simulink library "Ventilation"  (R2018b)
settings: Solver=ode45  StartTime=0.0  StopTime=10.0  RelTol=1e-3  EnableMultiTasking=on
libraries: carnot x4
settings Model: Creator=lena.frank  LastModifiedBy=drhf
settings DataIOCC: LimitDataPoints=on  SaveFormat=Array  SignalLoggingSaveFormat=ModelDataLogs
settings OptimizationCC: ExpressionDepthLimit=2147483647  LifeSpan=inf
settings DebuggingCC: UnderspecifiedInitializationDetection=Classic  MergeDetectMultiDrivingBlocksExec=none  SolverPrmCheckMsg=warning  FcnCallInpInsideContextMsg=warning  StateNameClashWarn=warning  SFUnexpectedBacktrackingDiag=warning  SFNoUnconditionalDefaultTransitionDiag=warning  SFExecutionAtInitializationDiag=none
settings HardwareCC: ProdBitPerPointer=32  ProdBitPerSizeT=32  ProdBitPerPtrDiffT=32  ProdLargestAtomicFloat=None  ProdIntDivRoundTo=Undefined  ProdEndianess=Unspecified  ProdWordSize=32  ProdHWDeviceType=32-bit Generic
settings ModelReferenceCC: PropagateSignalLabelsOutOfModel=off
settings SFSimCC: SimUseLocalCustomCode=off
settings RTWCC: RTWUseLocalCustomCode=off
settings CodeAppCC: StateflowObjectComments=on
settings GRTTargetCC: TargetLangStandard=C89/C90 (ANSI)  GeneratePreprocessorConditionals=Disable all  CombineOutputUpdateFcns=off  GRTInterface=on
settings ConfigComp: CovMetricSettings=dw  CovHtmlReporting=on  CovSaveCumulativeToWorkspaceVar=on  CovSaveSingleToWorkspaceVar=on  CovExternalEMLEnable=off

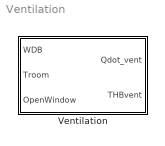
== system Ventilation ==
  Ventilation : Subsystem  mask(Ventilation with Heat Recovery and Window){Ahabit=50, Hroom=2, vent=0.6, rec=0.6, ppmCO2=400, ppmVOC=0, alpha=10, H=1, W=1, Nwin=1}
      mask prompts: Ahabit "A: heated surface of the house in m²"; Hroom "H: height of room in m"; vent "Air exchange rate (volume of house per hour) in 1/h"; rec "Heat recovery of ventilation in 0..1"; ppmCO2 "Concentration of CO2 in ppm"; ppmVOC "Concentration of VOC in ppm"; alpha "maximal opening angle (°)"; H "height of window (m)"; W "width of window (m)"; Nwin "Number of windows"
      mask help:
      | Model of a mechanical ventilation system with heat recovery and a ventilation with windows.
      | The model is suitable for the simple building model (/Load/Houses/House_simpe).
      mask init:
      | rec = max(0, min(1, rec));
      mask Help: web(fullfile(path_carnot('help'),'Ventilation.html'),'-helpbrowser')
      mask TypeOptions Ahabit: Ahabit/Value
      mask TypeOptions Hroom: Hroom/Gain
      mask TypeOptions vent: air_flow_rate/Gain
      mask TypeOptions rec: heatRecovery/Value
      mask TypeOptions ppmCO2: ppmCO2/Value
      mask TypeOptions ppmVOC: ppmVOC/Value
      mask TypeOptions alpha: Window_Ventilation/alpha
      mask TypeOptions H: Window_Ventilation/H
      mask TypeOptions W: Window_Ventilation/W
      mask TypeOptions Nwin: Window_Ventilation/Nwin
      mask DialogControl Container4 Prompt: Ventilation
      mask DialogControl Container5 Prompt: Windows
      mask Display:
      | plot(0,-0.2,1.2,1.2,[0.2 0.35], [0.8 0.7])
      | plot([0.35 0.65], [0.7 0.7])
      | plot([0.65 0.8], [0.7 0.8])
      | plot([0.65 0.8], [0.76 0.8])
      | plot([0.7 0.8], [0.65 0.8])
      | 
      | plot([0.2 0.35], [0.2 0.3])
      | plot([0.35 0.65], [0.3 0.3])
      | plot([0.65 0.8], [0.3 0.2])
      | plot([0.2 0.25], [0.2 0.32])
      | plot([0.2 0.35], [0.2 0.23])
      | 
      | plot ([0.45 0.45], [0 1])
      | plot ([0.55 0.55], [0 1])
      | 
      | plot ([0.45 0.55], [0.2 0.2])
      | plot ([0.45 0.55], [0.8 0.8])
      | 
      | plot ([0.45 0.55], [0 0.2])
      | plot ([0.45 0.55], [0.8 1])

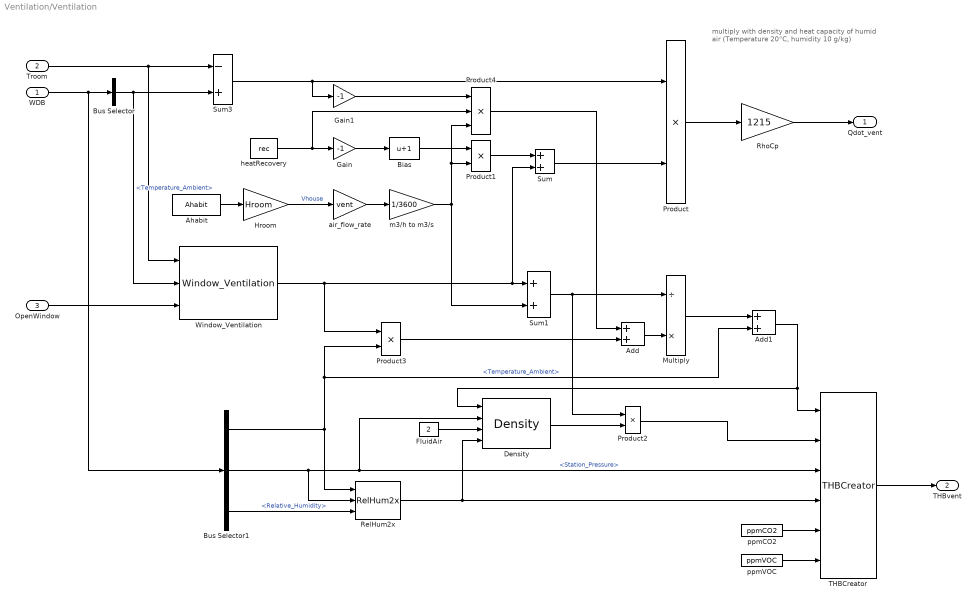
== system Ventilation/Ventilation ==
  note: multiply with density and
      | heat capacity of humid air
      | (Temperature 20°C, humidity 10 g/kg)
  WDB : Inport
  Troom : Inport  Port=2
  OpenWindow : Inport  Port=3
  Add : Sum
  Add1 : Sum
  Ahabit : Constant  Value=Ahabit
  Bias : Bias  Bias=1
  Bus Selector : BusSelector  OutputSignals=Temperature_Ambient
  Bus Selector1 : BusSelector  OutputSignals=Temperature_Ambient,Station_Pressure,Relative_Humidity
  Density : carnot/Basic/Material_Properties/Density  VariantControl=CarlibClassic  INPUTARGUMENTS=state variables (classic)  DEBUGLEVEL=DEBUGLEVEL  MAXTOTALWARNINGS=inf  MAXCONSECUTIVEWARNINGS=inf  WRITETOFILE=0  FILENAME='errors.txt'
      settings: SourceProductName=Carnot
  FluidAir : Constant  Value=2
  Gain : Gain  Gain=-1
  Gain1 : Gain  Gain=-1
  Hroom : Gain  Gain=Hroom
  Multiply : Product  Inputs=/*
  Product : Product  RndMeth=Zero
  Product1 : Product  Inputs=**  RndMeth=Zero
  Product2 : Product  RndMeth=Zero
  Product3 : Product  RndMeth=Zero
  Product4 : Product  Inputs=3  RndMeth=Zero
  RelHum2x : carnot/Basic/Material_Properties/RelHum2x
      settings: SourceProductName=Carnot
  RhoCp : Gain  Gain=1215  SaturateOnIntegerOverflow=on  OutDataTypeStr=Inherit: Same as input  ParamDataTypeStr=Inherit: Same as input
  Sum : Sum
  Sum1 : Sum
  Sum3 : Sum  Inputs=-+  SaturateOnIntegerOverflow=on  InputSameDT=on  OutDataTypeStr=Inherit: Same as first input
  THBCreator : carnot/Basic/Hydraulics/THBCreator  Inport_ID=off  Inport_T=on  Inport_mdot=on  Inport_p=on  Inport_type=off  Inport_mix=on  Inport_mix2=on  Inport_mix3=on  Inport_d=off  Inport_c=off  Inport_l=off  Inport_q=off  Inport_LH=off  Inport_H=off  ID=1  T=20  mdot=0  p=1e5  FluidType=2  FluidMix=0  FluidMix2=0  FluidMix3=0  d=1  c=0  l=0  q=0  LH=1  H=0  Annotation_ID=off  Annotation_T=off  Annotation_mdot=off  Annotation_p=off  Annotation_type=off  Annotation_mix=off  Annotation_mix2=off  Annotation_mix3=off  Annotation_d=off  Annotation_c=off  Annotation_l=off  Annotation_q=off  Annotation_LH=off  Annotation_H=off
      settings: SourceProductName=Carnot
  Window_Ventilation : carnot/Source/Ventilation/Window_Ventilation  alpha=alpha  H=H  W=W  Nwin=Nwin
      settings: SourceProductName=Carnot
  air_flow_rate : Gain  Gain=vent
  heatRecovery : Constant  Value=rec
  m3/h to m3/s : Gain  Gain=1/3600  SaturateOnIntegerOverflow=on  OutDataTypeStr=Inherit: Same as input  ParamDataTypeStr=Inherit: Same as input
  ppmCO2 : Constant  Value=ppmCO2
  ppmVOC : Constant  Value=ppmVOC
  Qdot_vent : Outport
  THBvent : Outport  Port=2
  wires:
  Gain/1 -> Bias/1
  heatRecovery/1 -> Product4/2, Gain/1
  OpenWindow/1 -> Window_Ventilation/3
  Troom/1 -> Window_Ventilation/1, Sum3/1
  m3/h to m3/s/1 -> Sum1/2, Product4/3, Product1/2
  WDB/1 -> Bus Selector/1, Bus Selector1/1
  Hroom/1 -> air_flow_rate/1  "Vhouse"
  Ahabit/1 -> Hroom/1
  Product/1 -> RhoCp/1
  Sum/1 -> Product/2
  THBCreator/1 -> THBvent/1
  Bus Selector/1 -> Sum3/2, Window_Ventilation/2  "<Temperature_Ambient>"
  Bus Selector1/1 -> Add1/2, Product3/2, RelHum2x/1  "<Temperature_Ambient>"
  Bus Selector1/2 -> THBCreator/3, Density/2, RelHum2x/2  "<Station_Pressure>"
  Bus Selector1/3 -> RelHum2x/3  "<Relative_Humidity>"
  RelHum2x/1 -> THBCreator/4, Density/4
  ppmCO2/1 -> THBCreator/5
  ppmVOC/1 -> THBCreator/6
  Product2/1 -> THBCreator/2
  air_flow_rate/1 -> m3/h to m3/s/1
  Density/1 -> Product2/2
  FluidAir/1 -> Density/3
  Window_Ventilation/1 -> Product3/1, Sum1/1, Sum/2
  RhoCp/1 -> Qdot_vent/1
  Product1/1 -> Sum/1
  Bias/1 -> Product1/1
  Sum1/1 -> Product2/1, Multiply/1
  Product3/1 -> Add/2
  Sum3/1 -> Product/1, Gain1/1
  Product4/1 -> Add/1
  Add/1 -> Multiply/2
  Multiply/1 -> Add1/1
  Add1/1 -> THBCreator/1, Density/1
  Gain1/1 -> Product4/1
